simulink model "TX_TUNE_DIGITALv2"  (R2024a)
settings: Solver=VariableStepAuto  StartTime=0.0  StopTime=1e-3  FixedStep=1e-9  RelTol=1e-3
values from neighbouring files (symbols this model uses):
  cnt_n_bits = 9    [TX_PM_MODEL_Setup.m]
  Cs = 12.5e-12    (= 1.25e-11)    [Oscillator_Setup.m]
  I0 = 100e-6    (= 0.0001)    [Oscillator_Setup.m]
  R = 0.2    [TX_PM_MODEL_Setup.m]
  Rf = 1e9    (= 1000000000)    [Oscillator_Setup.m]
  VDD = 5    [Oscillator_Setup.m]    (also in TX_PM_MODEL_Setup.m = 10)
  Vh = VDD - deltaVOSC    (= 4.5)    [Oscillator_Setup.m]
  Vl = deltaVOSC    (= 0.5)    [Oscillator_Setup.m]
undefined symbols (not defined in the file or in its folder): VDD_DRIVE
libraries: fl_lib x12, nesl_utility x7, MyLib x4, spsTriangleGeneratorLib x2, dspsigops x1, ee_lib x1
settings Model: Creator=cian.odonnell  LastModifiedBy=ciano
settings SolverCC: EnableFixedStepZeroCrossing=on

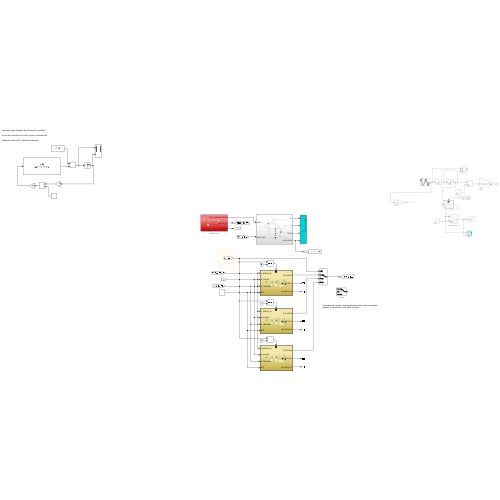
[thumbnail: Simulink's stored preview of the top-level diagram]
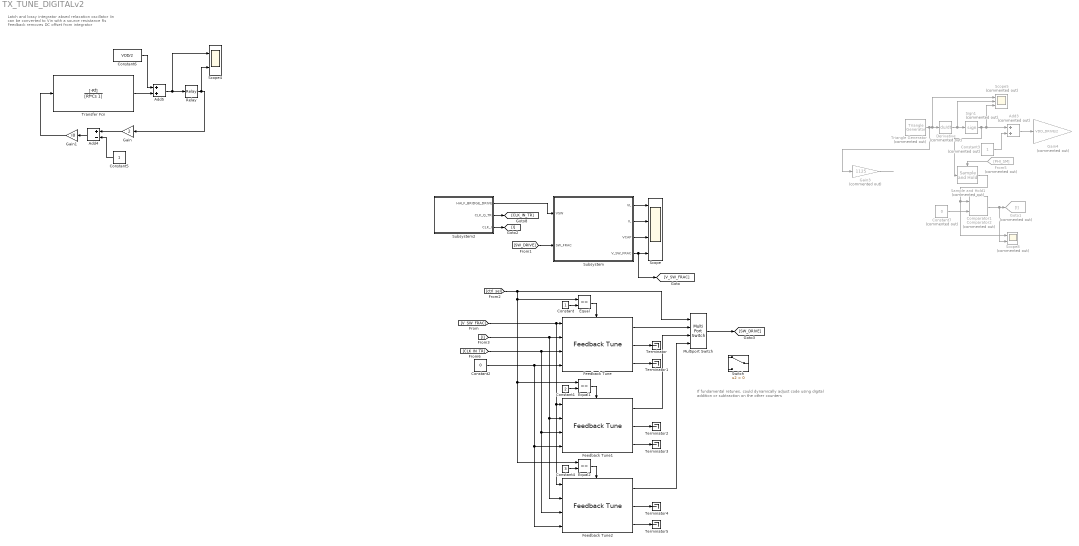
== system TX_TUNE_DIGITALv2 ==
  note: If fundamental retunes, could dynamically adjust code using digital
      | addition or subtraction on the other counters
  note: Latch and lossy integrator absed relaxation oscillator
      |
      | Iin can be converted to Vin with a source resistance Rs
      |
      | Feedback removes DC offset from integrator
  Add3 : Sum  Commented=on
  Add4 : Sum  Inputs=+-
  Add5 : Sum
  Comparator1 : MyLib/Comparator2  Commented=on  SystemSampleTime=-1  VariantActivationTime=update diagram  AllowFlexibleInterface=on  Latency=0  AutoFrameSizeCalculation=off
  Constant : Constant
  Constant1 : Constant  Value=2
  Constant2 : Constant  Value=0
  Constant3 : Constant  Commented=on
  Constant4 : Constant  Value=3
  Constant5 : Constant
  Constant6 : Constant  Value=VDD/2
  Constant7 : Constant  Commented=on  Value=0
  Derivative : Derivative  Commented=on
  Equal : RelationalOperator  Operator===  OutDataTypeStr=boolean  RndMeth=Simplest  InputSameDT=off
  Equal1 : RelationalOperator  Operator===  OutDataTypeStr=boolean  RndMeth=Simplest  InputSameDT=off
  Equal2 : RelationalOperator  Operator===  OutDataTypeStr=boolean  RndMeth=Simplest  InputSameDT=off
  Feedback Tune : MyLib/Feedback Tune  SystemSampleTime=-1  VariantActivationTime=update diagram  AllowFlexibleInterface=on  Latency=0  AutoFrameSizeCalculation=off
  Feedback Tune1 : MyLib/Feedback Tune  SystemSampleTime=-1  VariantActivationTime=update diagram  AllowFlexibleInterface=on  Latency=0  AutoFrameSizeCalculation=off
  Feedback Tune2 : MyLib/Feedback Tune  SystemSampleTime=-1  VariantActivationTime=update diagram  AllowFlexibleInterface=on  Latency=0  AutoFrameSizeCalculation=off
  From5 : From  Commented=on  GotoTag=PHI_SM
  Gain : Gain  Gain=2
  Gain1 : Gain  Gain=I0
  Gain3 : Gain  Commented=on  Gain=1125
  Gain4 : Gain  Commented=on  Gain=VDD_DRIVE/2
  Goto1 : Goto  Commented=on  GotoTag=I
  Multiport Switch : MultiPortSwitch  SaturateOnIntegerOverflow=off  InputSameDT=off
  Relay : Relay  OnSwitchValue=Vh  OffSwitchValue=Vl
  Sample and Hold1 : dspsigops/Sample and Hold  Commented=on  trig=Either edge  initCond=0  latchinput=off
  Scope : Scope  NumInputPorts=4
  Scope4 : Scope  NumInputPorts=2
  Scope5 : Scope  Commented=on  NumInputPorts=3
  Scope8 : Scope  Commented=on  NumInputPorts=2
  Sign1 : Signum  Commented=on
  Subsystem : Subsystem
  Subsystem2 : Subsystem
  Switch : Switch  Criteria=u2 > Threshold  SaturateOnIntegerOverflow=off  InputSameDT=off
  Terminator{,1..5} (6 alike) : Terminator
  Transfer Fcn : TransferFcn  Numerator=[-Rf]  Denominator=[Rf*Cs 1]
  Triangle Generator : spsTriangleGeneratorLib/Triangle Generator  Commented=on  Freq=fin  Phase=90  Ts=0
  wires:
  Add5/1 -> Scope4/1, Relay/1
  Transfer Fcn/1 -> Add5/2
  Gain1/1 -> Transfer Fcn/1
  Add4/1 -> Gain1/1
  Gain/1 -> Add4/1
  Constant5/1 -> Add4/2
  Constant6/1 -> Add5/1
  Relay/1 -> Gain/1, Scope4/2
  Subsystem/1(VL) -> Scope/1
  Subsystem/2(IL) -> Scope/2
  Subsystem/3(VCAP) -> Scope/3
  Constant2/1 -> Feedback Tune/4, Feedback Tune2/4, Feedback Tune1/4
  Subsystem/4(V_SW_FRAC) -> [V_SW_FRAC], Scope/4
  Feedback Tune/2 -> Terminator/1
  Feedback Tune/3 -> Terminator1/1
  [I] -> Feedback Tune/2, Feedback Tune2/2, Feedback Tune1/2
  [CLK_IN_TR] -> Feedback Tune2/3, Feedback Tune1/3, Feedback Tune/3
  Subsystem2/2(CLK_Q_TR) -> [CLK_IN_TR]
  Subsystem2/3(CLK_I) -> [I]
  Comparator1/1 -> Scope8/2, Goto1/1
  Add3/1 -> Gain4/1
  Derivative/1 -> Sign1/1, Scope5/2
  Constant3/1 -> Add3/2
  Sample and Hold1/1 -> Comparator1/1, Scope8/1
  From5/1 -> Sample and Hold1/Trigger
  Constant7/1 -> Comparator1/2
  Triangle Generator/1 -> Scope5/1, Derivative/1, Gain3/1
  Sign1/1 -> Sample and Hold1/1, Add3/1, Scope5/3
  Gain3/1 -> ?
  Subsystem2/1(HALF_BRIDGE_DRIVE) -> Subsystem/1(VSW)
  Feedback Tune/1 -> Multiport Switch/2
  [V_SW_FRAC] -> Feedback Tune/1, Feedback Tune2/1, Feedback Tune1/1
  Feedback Tune1/3 -> Terminator3/1
  Feedback Tune1/2 -> Terminator2/1
  Feedback Tune2/2 -> Terminator4/1
  Feedback Tune2/3 -> Terminator5/1
  Feedback Tune1/1 -> Multiport Switch/3
  Feedback Tune2/1 -> Multiport Switch/4
  Multiport Switch/1 -> [SW_DRIVE]
  [SW_DRIVE] -> Subsystem/2(SW_FRAC)
  Equal/1 -> Feedback Tune/Enable
  Constant/1 -> Equal/2
  Equal1/1 -> Feedback Tune1/Enable
  Constant1/1 -> Equal1/2
  Equal2/1 -> Feedback Tune2/Enable
  Constant4/1 -> Equal2/2
  [ctrl_sel] -> Equal2/1, Equal1/1, Equal/1, Multiport Switch/1

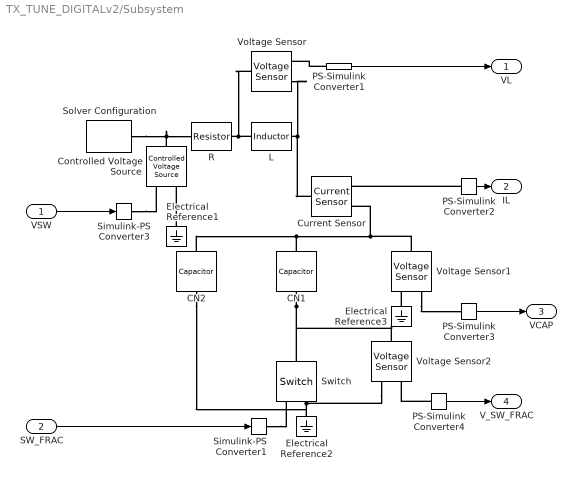
== system TX_TUNE_DIGITALv2/Subsystem ==
  VSW : Inport
  SW_FRAC : Inport  Port=2
  CN1 : fl_lib/Electrical/Electrical Elements/Capacitor  c=3e-9 F  r=1e-6 Ohm  g=0 1/Ohm  i_specify=off  i_priority=None  i=0 A  i_nominal_specify=off  i_nominal_value=1  i_nominal_unit=A  v_specify=off  v_priority=None  v=0 V  v_nominal_specify=off  v_nominal_value=1  v_nominal_unit=V  vc_specify=off  vc_priority=High  vc=0 V  vc_nominal_specify=off  vc_nominal_value=1  vc_nominal_unit=V
  CN2 : fl_lib/Electrical/Electrical Elements/Capacitor  c=3e-9 F  r=1e-6 Ohm  g=0 1/Ohm  i_specify=off  i_priority=None  i=0 A  i_nominal_specify=off  i_nominal_value=1  i_nominal_unit=A  v_specify=off  v_priority=None  v=0 V  v_nominal_specify=off  v_nominal_value=1  v_nominal_unit=V  vc_specify=off  vc_priority=High  vc=0 V  vc_nominal_specify=off  vc_nominal_value=1  vc_nominal_unit=V
  Controlled Voltage Source : fl_lib/Electrical/Electrical Sources/Controlled Voltage Source
  Current Sensor : fl_lib/Electrical/Electrical Sensors/Current Sensor
  Electrical Reference1 : fl_lib/Electrical/Electrical Elements/Electrical Reference
  Electrical Reference2 : fl_lib/Electrical/Electrical Elements/Electrical Reference
  Electrical Reference3 : fl_lib/Electrical/Electrical Elements/Electrical Reference
  L : ee_lib/Passive/Inductor  l=L H  enable_L_tol=ee.enum.toleranceApplication.none  L_tol=20  tol_distribution=ee.enum.toleranceDistribution.uniform  nSigma=4  r=0 Ohm  g=1e-9 1/Ohm  enable_operating_limits=ee.enum.enable.no  operating_limit_action=ee.enum.passive.reportOpLim.warn  max_working_current=1 A  power_rating=1 W  enable_faults=ee.enum.enable.no  fault_action=simscape.enum.assert.action.none  lambdaPercent=50  k_faulted=0.9999  turnsShort=ee.enum.passive.inductor.turnsShortOption.no  openCct=ee.enum.enable.no  groundShort=ee.enum.passive.inductor.groundShortOption.no  groundShortG=0 1/Ohm  tau_fault=1e-3 s  fault_trigger=ee.enum.faults.faultTrigger.temporal  t_fault=1 s  max_permissible_voltage=100 V  n_fail_on_voltage=1  max_permissible_current=1 A  t_fail_on_current=1 s  i_L_specify=off  i_L_priority=High  i_L=0 A  i_L_nominal_specify=off  i_L_nominal_value=1  i_L_nominal_unit=A  faulted_specify=off  faulted_priority=None  faulted=0
  PS-Simulink Converter{1..4} (4 alike) : nesl_utility/PS-Simulink Converter  PhysicalDomain=network_engine_domain  SubClassName=ps_output  LeftPortType=input  RightPortType=output  PseudoPeriodic=off  Frequencies=[]  VectorFormat=inherit  Unit=inherit  AffineConversion=off
  R : fl_lib/Electrical/Electrical Elements/Resistor  R=R Ohm  i_specify=off  i_priority=None  i=0 A  i_nominal_specify=off  i_nominal_value=1  i_nominal_unit=A  v_specify=off  v_priority=None  v=0 V  v_nominal_specify=off  v_nominal_value=1  v_nominal_unit=V
  Simulink-PS Converter1 : nesl_utility/Simulink-PS Converter  PhysicalDomain=network_engine_domain  SubClassName=ps_input  LeftPortType=input  RightPortType=output  PseudoPeriodic=off  Frequencies=[]  NoiseDistribution=none  NoiseParameters=[]  Unit=1  AffineConversion=off  FilteringAndDerivatives=provide  SimscapeFilterOrder=1  InputFilterTimeConstant=0.001  UdotUserProvided=0
  Simulink-PS Converter3 : nesl_utility/Simulink-PS Converter  PhysicalDomain=network_engine_domain  SubClassName=ps_input  LeftPortType=input  RightPortType=output  PseudoPeriodic=off  Frequencies=[]  NoiseDistribution=none  NoiseParameters=[]  Unit=1  AffineConversion=off  FilteringAndDerivatives=provide  SimscapeFilterOrder=1  InputFilterTimeConstant=0.001  UdotUserProvided=0
  Solver Configuration : nesl_utility/Solver Configuration  PhysicalDomain=network_engine_domain  SubClassName=solver  LeftPortType=input  RightPortType=generic  Tones=[]  Harmonics=[]  SimulateNoise=off  Profile=off  UseLocalSampling=off  EnableSwitchedLinearOptims=on  FrequencyDomain=off  UseCCode=off  RelTol=0.001  AbsTol=0.001  MinStep=1e-09  ToWorkspace=off  RevertToSquareIcSolve=off  NumHomotopyIterations=100  PhasorMode=off  PhasorModeNumHarmonics=1  ConsistencySolver=NEWTON_XTOL_AFTER_FTOL  IndexReductionMethod=DerivativeReplacement  DoDC=off  ResidualTolerance=1e-09  ConsistencyTolSource=GLOBAL  ConsistencyAbsTol=0.001  ConsistencyRelTol=0.001  ConsistencyTolFactor=0.001  UseLocalSolver=off  LocalSolverChoice=NE_BACKWARD_EULER_ADVANCER  ResolveIndetEquations=on  FunctionEvalNumThread=1  LocalSolverSampleTime=0.001  DoFixedCost=off  MaxNonlinIter=3  MaxModeIter=2  ComputeImpulses=off  ImpulseIterations=2  LinearAlgebra=auto  LinearAlgebraNumThread=0  EquationFormulation=NE_TIME_EF  DelaysMemoryBudget=1024  AutomaticFiltering=on  FilteringTimeConstant=0.001  PartitionStorageMethod=AS_NEEDED  PartitionMemoryBudget=1024  PartitionMethod=ROBUST  MultibodyUseLocalSolver=off  MultibodyLocalSolverChoice=ODE1  MultibodyLocalSolverSampleTime=0.001
  Switch : fl_lib/Electrical/Electrical Elements/Switch  R_closed=0.01 Ohm  G_open=1e-8 1/Ohm  Threshold=0.5  i_specify=off  i_priority=None  i=0 A  i_nominal_specify=off  i_nominal_value=1  i_nominal_unit=A  v_specify=off  v_priority=None  v=0 V  v_nominal_specify=off  v_nominal_value=1  v_nominal_unit=V
  Voltage Sensor : fl_lib/Electrical/Electrical Sensors/Voltage Sensor
  Voltage Sensor1 : fl_lib/Electrical/Electrical Sensors/Voltage Sensor
  Voltage Sensor2 : fl_lib/Electrical/Electrical Sensors/Voltage Sensor
  VL : Outport
  IL : Outport  Port=2
  VCAP : Outport  Port=3
  V_SW_FRAC : Outport  Port=4
  wires:
  PS-Simulink Converter3/1 -> VCAP/1
  SW_FRAC/1 -> Simulink-PS Converter1/1
  PS-Simulink Converter2/1 -> IL/1
  PS-Simulink Converter4/1 -> V_SW_FRAC/1
  VSW/1 -> Simulink-PS Converter3/1
  PS-Simulink Converter1/1 -> VL/1
  connections:
  Current Sensor/LConn1 -- Voltage Sensor/RConn2 -- L/RConn1
  Electrical Reference1/LConn1 -- Controlled Voltage Source/RConn2
  Voltage Sensor1/RConn1 -- PS-Simulink Converter3/LConn1
  Electrical Reference3/LConn1 -- Voltage Sensor1/RConn2
  CN1/RConn1 -- Voltage Sensor2/LConn1 -- Switch/LConn1
  Simulink-PS Converter3/RConn1 -- Controlled Voltage Source/RConn1
  CN1/LConn1 -- Voltage Sensor1/LConn1 -- Current Sensor/RConn2 -- CN2/LConn1
  PS-Simulink Converter2/LConn1 -- Current Sensor/RConn1
  PS-Simulink Converter1/LConn1 -- Voltage Sensor/RConn1
  Electrical Reference2/LConn1 -- CN2/RConn1 -- Switch/RConn2 -- Voltage Sensor2/RConn2
  Simulink-PS Converter1/RConn1 -- Switch/RConn1
  PS-Simulink Converter4/LConn1 -- Voltage Sensor2/RConn1
  L/LConn1 -- Voltage Sensor/LConn1 -- R/RConn1
  Controlled Voltage Source/LConn1 -- R/LConn1 -- Solver Configuration/RConn1

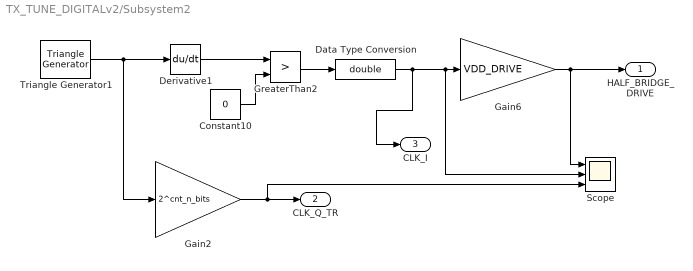
== system TX_TUNE_DIGITALv2/Subsystem2 ==
  Constant10 : Constant  Value=0
  Data Type Conversion : DataTypeConversion  OutDataTypeStr=double  SaturateOnIntegerOverflow=off  RndMeth=Floor
  Derivative1 : Derivative
  Gain2 : Gain  Gain=2^cnt_n_bits
  Gain6 : Gain  Gain=VDD_DRIVE
  GreaterThan2 : RelationalOperator  Operator=>  OutDataTypeStr=boolean  RndMeth=Simplest  InputSameDT=off
  Scope : Scope  NumInputPorts=3
  Triangle Generator1 : spsTriangleGeneratorLib/Triangle Generator  Freq=fin  Phase=90  Ts=0
  HALF_BRIDGE_DRIVE : Outport
  CLK_Q_TR : Outport  Port=2
  CLK_I : Outport  Port=3
  wires:
  Triangle Generator1/1 -> Derivative1/1, Gain2/1
  Gain6/1 -> Scope/1, HALF_BRIDGE_DRIVE/1
  Gain2/1 -> Scope/3, CLK_Q_TR/1
  Derivative1/1 -> GreaterThan2/1
  GreaterThan2/1 -> Data Type Conversion/1
  Constant10/1 -> GreaterThan2/2
  Data Type Conversion/1 -> CLK_I/1, Scope/2, Gain6/1
